simulink model "rf_boiler_open_loop"  (R2017a)
settings: Solver=FixedStepAuto  StartTime=0.0  StopTime=simTime  FixedStep=Dt  RelTol=1e-3  EnableMultiTasking=on
values from neighbouring files (symbols this model uses):
  D0 = 35.783396242    [cic2017_fase1_boiler.mat]    (also in compare_rf_boiler.m = 35.7834; control_Caldera_3004.m = 35.7834; mpcGASimulink_2205_dummy.m = 35.7834; mpc_design_parameters_0206.mat = 35.7834)
  Dt = 1    [compare_rf_boiler.m]    (also in control_Caldera_3004.m = 0.5; mpcBoiler_0206.m; mpcBoiler_2805.m; mpcBoiler_closed_loop_0206.m)
  make = makeMatrix(m,:)    [compare_rf_boiler.m]    (also in mpcGASimulink_2205_dummy.m = [1 0 1 1]; rf_boiler_simulateScript.m; simScript.m = [1 0 1 1]; testBigData.m)
  maxDDelay = maxDelay(3)    [compare_rf_boiler.m]    (also in mpcGASimulink_2205_dummy.m = max(max(nc)); mpc_design_parameters_0206.mat = 2; mpc_design_parameters_0606.mat = 2; mpc_design_parameters_0706.mat = 2)
  maxUDelay = maxDelay(2)    [compare_rf_boiler.m]    (also in mpcGASimulink_2205_dummy.m = max(max(nb)); mpc_design_parameters_0206.mat = 2; mpc_design_parameters_0606.mat = 2; mpc_design_parameters_0706.mat = 2)
  maxYDelay = maxDelay(1)    [compare_rf_boiler.m]    (also in mpcGASimulink_2205_dummy.m = max(na); mpc_design_parameters_0206.mat = 4; mpc_design_parameters_0606.mat = 4; mpc_design_parameters_0706.mat = 4)
  na = [delayYMatrix(2,2);delayYMatrix(2,2);delayYMatrix(3,3)]    [mpcGASimulink_2205_dummy.m]    (also in mpc_design_parameters_0206.mat = [4 4 4]; mpc_design_parameters_0606.mat = [4 4 4]; mpc_design_parameters_0706.mat = [4 4 4]; mpc_design_parameters_2805.mat = [4 3 4])
  nb = delayUMatrix(:,2:end)    [mpcGASimulink_2205_dummy.m]    (also in mpc_design_parameters_0206.mat = [1  1  1; 2  2  2; 2  2  2]; mpc_design_parameters_0606.mat = [1  1  1; 2  2  2; 2  2  2]; mpc_design_parameters_0706.mat = [1  1  1; 2  2  2; 2  2  2]; mpc_design_parameters_2805.mat = [1  1  1; 1  1  1; 1  2  1])
  nc = delayUMatrix(:,1)    [mpcGASimulink_2205_dummy.m]    (also in mpc_design_parameters_0206.mat = [1 2 2]; mpc_design_parameters_0606.mat = [1 2 2]; mpc_design_parameters_0706.mat = [1 2 2]; mpc_design_parameters_2805.mat = [1 1 2])
  nPredictors = [8 12 12]    [compare_rf_boiler.m]    (also in mpcGASimulink_2205_dummy.m = 10*ones(1,3); mpc_design_parameters_0206.mat; mpc_design_parameters_0606.mat; mpc_design_parameters_0706.mat)
  nTrees = ones(1,numCV)*100    [compare_rf_boiler.m]    (also in mpcGASimulink_2205_dummy.m = ones(1,3)*100; mpc_design_parameters_0206.mat = [100 100 100]; mpc_design_parameters_0606.mat = [100 100 100]; mpc_design_parameters_0706.mat = [100 100 100])
  U0 = [32.9815865199 46.2282063472 25.3416381967]    [cic2017_fase1_boiler.mat]    (also in compare_rf_boiler.m = [32.9816   46.2282   25.3416]; control_Caldera_3004.m = [32.9816   46.2282   25.3416]; mpcGASimulink_2205_dummy.m = [32.9816   46.2282   25.3416]; mpc_design_parameters_0206.mat = [32.9816 46.2282 25.3416])
  Y0 = [41.4119839556 28.7552838432 38.6036799989]    [cic2017_fase1_boiler.mat]    (also in compare_rf_boiler.m = [41.4120   28.7553   38.6037]; control_Caldera_3004.m = [41.4120   28.7553   38.6037]; mpcGASimulink_2205_dummy.m = [41.4120   28.7553   38.6037]; mpc_design_parameters_0206.mat = [41.412 28.7553 38.6037])
settings Model: Creator=Pablo Diaz  LastModifiedBy=Pablo Diaz
settings OptimizationCC: LifeSpan=inf
settings DebuggingCC: SFUnexpectedBacktrackingDiag=warning  SFNoUnconditionalDefaultTransitionDiag=warning  SFExecutionAtInitializationDiag=none
settings GRTTargetCC: TargetLangStandard=C89/C90 (ANSI)
settings ConfigComp: CovMetricSettings=dw  CovHtmlReporting=on  CovSaveCumulativeToWorkspaceVar=on  CovSaveSingleToWorkspaceVar=on  CovExternalEMLEnable=off

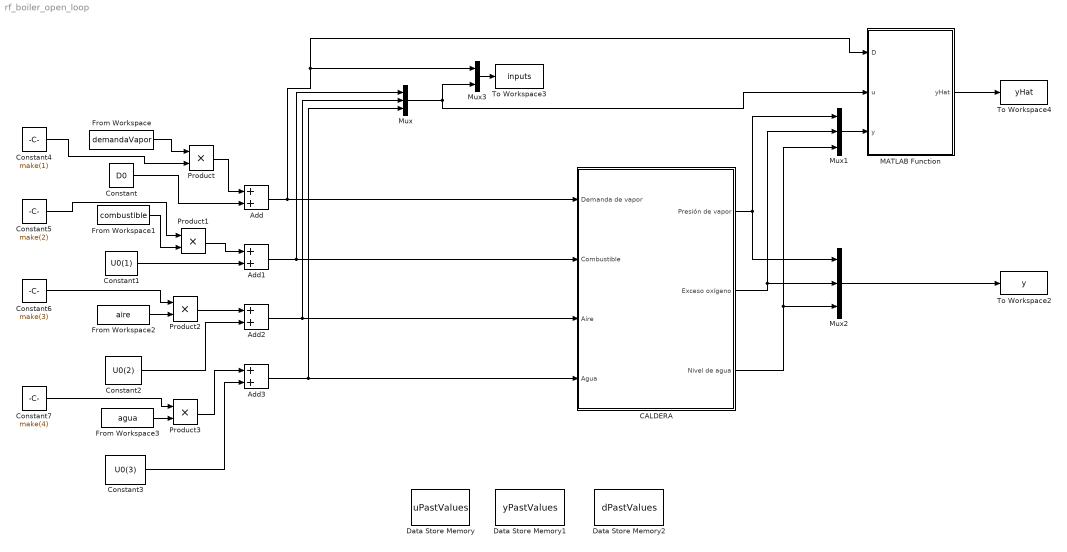
== system rf_boiler_open_loop ==
  Add{,1..3} (4 alike) : Sum
  CALDERA : Subsystem
  Constant : Constant  Value=D0
  Constant1 : Constant  Value=U0(1)
  Constant2 : Constant  Value=U0(2)
  Constant3 : Constant  Value=U0(3)
  Constant4 : Constant  Value=make(1)
  Constant5 : Constant  Value=make(2)
  Constant6 : Constant  Value=make(3)
  Constant7 : Constant  Value=make(4)
  Data Store Memory : DataStoreMemory  DataStoreName=uPastValues  ReadBeforeWriteMsg=warning  WriteAfterWriteMsg=warning  WriteAfterReadMsg=warning  InitialValue=[U0]'*ones(1,maxUDelay);  VectorParams1D=off  ShowAdditionalParam=off  OutDataTypeStr=double
  Data Store Memory1 : DataStoreMemory  DataStoreName=yPastValues  ReadBeforeWriteMsg=warning  WriteAfterWriteMsg=warning  WriteAfterReadMsg=warning  InitialValue=Y0'*ones(1,maxYDelay)  VectorParams1D=off  ShowAdditionalParam=off  OutDataTypeStr=double
  Data Store Memory2 : DataStoreMemory  DataStoreName=dPastValues  ReadBeforeWriteMsg=warning  WriteAfterWriteMsg=warning  WriteAfterReadMsg=warning  InitialValue=D0'*ones(1,maxDDelay)  VectorParams1D=off  ShowAdditionalParam=off  OutDataTypeStr=double
  From Workspace : FromWorkspace  VariableName=demandaVapor  SampleTime=Dt
  From Workspace1 : FromWorkspace  VariableName=combustible  SampleTime=Dt
  From Workspace2 : FromWorkspace  VariableName=aire  SampleTime=Dt
  From Workspace3 : FromWorkspace  VariableName=agua  SampleTime=Dt
  MATLAB Function : MATLAB Function  TreatAsAtomicUnit=on
  Mux : Mux  Inputs=3
  Mux1 : Mux  Inputs=3
  Mux2 : Mux  Inputs=3
  Mux3 : Mux  Inputs=2
  Product{,1..3} (4 alike) : Product
  To Workspace2 : ToWorkspace  VariableName=y  SaveFormat=Structure With Time  SampleTime=-1
  To Workspace3 : ToWorkspace  VariableName=inputs  SaveFormat=Structure With Time  SampleTime=-1
  To Workspace4 : ToWorkspace  VariableName=yHat  SaveFormat=Structure With Time  SampleTime=-1
  wires:
  CALDERA/2(Exceso oxígeno) -> Mux2/2, Mux1/2
  From Workspace/1 -> Product/1
  Constant/1 -> Add/2
  From Workspace1/1 -> Product1/2
  Constant1/1 -> Add1/2
  From Workspace2/1 -> Product2/2
  Add2/1 -> Mux/2, CALDERA/3(Aire)
  Constant2/1 -> Add2/2
  From Workspace3/1 -> Product3/2
  Add3/1 -> Mux/3, CALDERA/4(Agua)
  Constant3/1 -> Add3/2
  Constant4/1 -> Product/2
  Product/1 -> Add/1
  Constant5/1 -> Product1/1
  Product1/1 -> Add1/1
  Constant6/1 -> Product2/1
  Product2/1 -> Add2/1
  Product3/1 -> Add3/1
  Constant7/1 -> Product3/1
  Add1/1 -> Mux/1, CALDERA/2(Combustible)
  Add/1 -> MATLAB Function/1(D), Mux3/1, CALDERA/1(Demanda de vapor)
  Mux/1 -> Mux3/2, MATLAB Function/2(u)
  CALDERA/1(Presión de vapor) -> Mux2/1, Mux1/1
  MATLAB Function/1(yHat) -> To Workspace4/1
  CALDERA/3(Nivel de agua) -> Mux1/3, Mux2/3
  Mux1/1 -> MATLAB Function/3(y)
  Mux2/1 -> To Workspace2/1
  Mux3/1 -> To Workspace3/1

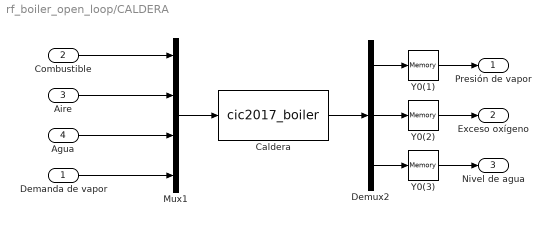
== system rf_boiler_open_loop/CALDERA ==
  Demanda de vapor : Inport
  Combustible : Inport  Port=2
  Aire : Inport  Port=3
  Agua : Inport  Port=4
  Caldera : S-Function  FunctionName=cic2017_boiler  Parameters=Y0,[U0 D0]  SFunctionDeploymentMode=off  EnableBusSupport=off
  Demux2 : Demux  Outputs=3
  Mux1 : Mux
  Y0(1) : Memory  X0=Y0(1)
  Y0(2) : Memory  X0=Y0(2)
  Y0(3) : Memory  X0=Y0(3)
  Presión de vapor : Outport
  Exceso oxígeno : Outport  Port=2
  Nivel de agua : Outport  Port=3
  wires:
  Caldera/1 -> Demux2/1
  Aire/1 -> Mux1/2
  Agua/1 -> Mux1/3
  Demanda de vapor/1 -> Mux1/4
  Combustible/1 -> Mux1/1
  Mux1/1 -> Caldera/1
  Demux2/1 -> Y0(1)/1
  Demux2/2 -> Y0(2)/1
  Demux2/3 -> Y0(3)/1
  Y0(1)/1 -> Presión de vapor/1
  Y0(2)/1 -> Exceso oxígeno/1
  Y0(3)/1 -> Nivel de agua/1

== matlab function rf_boiler_open_loop/MATLAB Function ==
  data: D input; yHat output size=[3 1]; u input; y input; nTrees parameter; nPredictors parameter; na parameter; nb parameter; nc parameter; yPastValues data_store_memory; uPastValues data_store_memory; dPastValues data_store_memory
function yHat = rf_plant_model(D, u, y,...
                nTrees, nPredictors, na, nb, nc)
coder.extrinsic('predictRF_Y1_mex');
coder.extrinsic('predictRF_Y2_mex');
coder.extrinsic('predictRF_Y3_mex');
global yPastValues
global uPastValues
global dPastValues
% u: vector containing [dv mv(1) mv(2) mv(3)];0
% y: vector containing [y(1) y(2) y(3)]

%   - nc: n*d containing order of DV delay for each CV
[n,~] = size(na);
[n,m] = size(nb);
[n,d] = size(nc);
yHat = zeros(n,1);
% Refresh past values for prediction in t+tau_R
yPastValues(:,2:end) = yPastValues(:,1:end-1);
yPastValues(:,1) = y(:);

dPastValues(:,2:end) = dPastValues(:,1:end-1);
dPastValues(:,1) = D(:);

uPastValues(:,2:end) = uPastValues(:,1:end-1);
uPastValues(:,1) = u(:);

predictorArray = generate_predictor_array_OL(yPastValues,uPastValues,dPastValues,...
                                            na,nb,nc);
for cv = 1:n
    % Predict
%     p = na(cv)+sum(nb(cv,:))+m+nc(cv,:)+d;
    p = na(cv)+sum(nb(cv,:))+nc(cv,:);
    if nTrees(cv) ~= 100
       error('Number of trees is %d in hardcoded function. Different from: %d',100,nTrees(cv)); 
    end
    if nPredictors(cv) ~= p
       error('Number of predictors is %d in hardcoded function. Different from: %d',p,nPredictors(cv)); 
    end
    X = predictorArray(1:p,cv);
    switch cv
        case 1
            yHat(cv) = predictRF_Y1_mex(X,nTrees(cv),p);
        case 2
            yHat(cv) = predictRF_Y2_mex(X,nTrees(cv),p);
        case 3
            yHat(cv) = predictRF_Y3_mex(X,nTrees(cv),p);
    end
end
